simulink model "fcev_model"  (R2023a)
settings: Solver=VariableStepAuto  StartTime=0.0  StopTime=2474  RelTol=1e-3
model workspace (MAT data in the model file):
  N_P0 = 3
values from neighbouring files (symbols this model uses):
  drive_Ki = 1    [fcev_model_parameters.m]
  drive_Kp = 20    [fcev_model_parameters.m]
  env_ambtemp_C = 25    [fcev_model_parameters.m]
  env_grade = 0    [fcev_model_parameters.m]
  env_windx_mps = 0    [fcev_model_parameters.m]
  mot_gearratio = 3.2    [fcev_model_parameters.m]
  mot_maxtrq_Nm = [85, 85, 85, 80, 70, 55, 30]    [fcev_model_parameters.m]
  mot_rotspd_radps = [0, 100, 200, 300, 400, 500, 600]    [fcev_model_parameters.m]
  mot_tirerad_m = 0.31    [fcev_model_parameters.m]
  tank_engydensH2_MJpkg = 120    [fcev_model_parameters.m]
  tank_fccurr_A = -20    [fcev_model_parameters.m]
  tank_fceff = 0.55    [fcev_model_parameters.m]
  tank_Pstart_bar = 350    [fcev_model_parameters.m]
  tank_Rconst = 4.124    [fcev_model_parameters.m]
  tank_temp_K = 298    [fcev_model_parameters.m]
  tank_vol_L = 7    [fcev_model_parameters.m]
libraries: nesl_utility x7, sdl_lib x6, autolibshared x2, fl_lib x2, autolibdatasheetbattery x1, autolibmappedmotor x1
settings Model: Creator=connl  LastModifiedBy=connl
settings SolverCC: MaxConsecutiveMinStep=5  DaesscMode=Robust  SolverResetMethod=Robust
settings DebuggingCC: AlgebraicLoopMsg=none

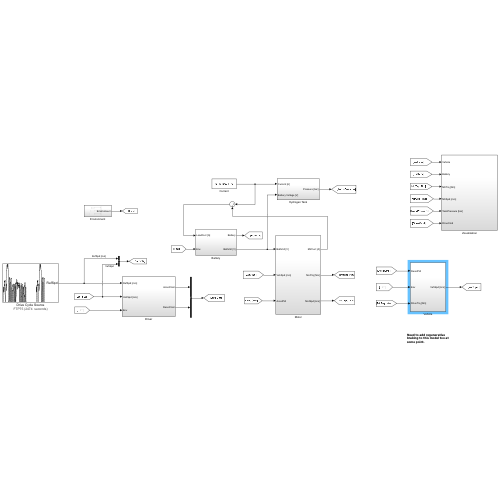
[thumbnail: Simulink's stored preview of the top-level diagram]
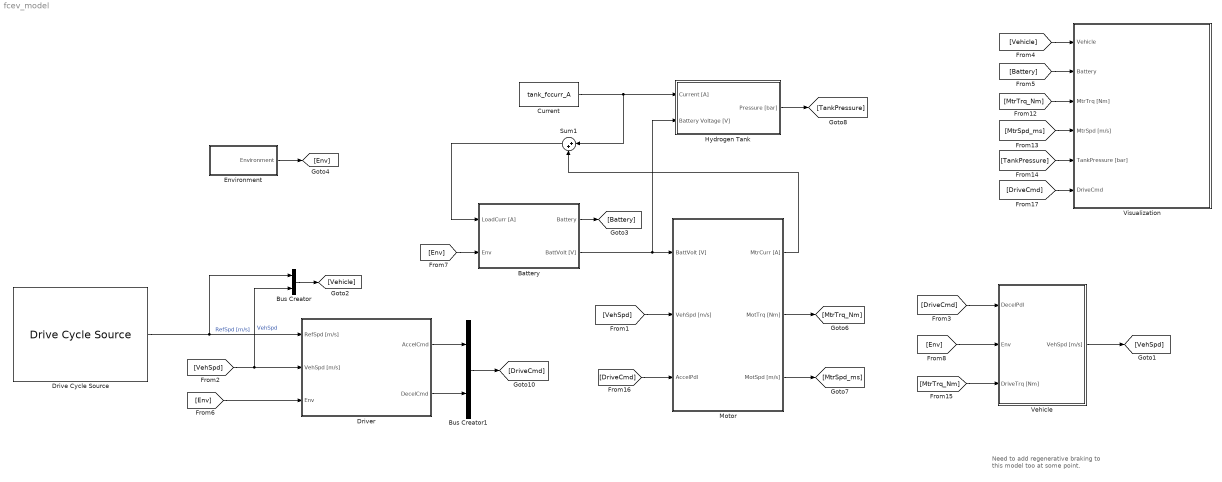
== system fcev_model ==
  note: Need to add regenerative braking to this model too at some point.
  Battery : Subsystem
  Bus Creator : BusCreator  Inputs=2
  Bus Creator1 : BusCreator  Inputs=2
  Current : Constant  Value=tank_fccurr_A
  Drive Cycle Source : autolibshared/Drive Cycle Source  cycleVar=FTP75  fileVar=cycleFTP75.mat  tfinal="2474  seconds"  cycleRepeat=off  outAccPort=off  outGearPort=off  gearList=No gear data  t_wot1=5  xdot_woto=0  xdot_wot1=30  t_wot2=20  xdot_wot2=0  t_wotend=30  srcUnit=m/s  outUnit=m/s  srcAccUnit=m/s/s  outAccUnit=m/s^2  dt=0  aMode=1  faultOption=off  velBnd=2  velBndUnit=mph  inUnit=m/s  timeBnd=1  failOption=off  stopSim=off  maxFaultCnt=10  maxFaultTime=2  maxTotFaultTime=15  traceOption=off  dtTrace=1  traceWindow=10  lastDCname=FTP75  lastOutUnit=mph  lastDT=0  lastTB=1  lastSB=2  forceCalcBound=off
  Driver : Subsystem
  Environment : Subsystem
  Hydrogen Tank : Subsystem
  Motor : Subsystem
  Sum1 : Sum  Inputs=|++
  Vehicle : Subsystem
  Visualization : Subsystem
  wires:
  Drive Cycle Source/1 -> Driver/1(RefSpd [m/s]), Bus Creator/1  "RefSpd [m/s]"
  Battery/2(BattVolt [V]) -> Motor/1(BattVolt [V]), Hydrogen Tank/2(Battery Voltage [V])
  [VehSpd] -> Motor/2(VehSpd [m/s])
  [VehSpd] -> Driver/2(VehSpd [m/s]), Bus Creator/2  "VehSpd"
  [DriveCmd] -> Vehicle/1(DecelPdl)
  Vehicle/1(VehSpd [m/s]) -> [VehSpd]
  Bus Creator/1 -> [Vehicle]
  [Vehicle] -> Visualization/1(Vehicle)
  [Battery] -> Visualization/2(Battery)
  Environment/1(Environment) -> [Env]
  Battery/1(Battery) -> [Battery]
  Driver/2(DecelCmd) -> Bus Creator1/2
  [Env] -> Battery/2(Env)
  [Env] -> Driver/3(Env)
  [Env] -> Vehicle/2(Env)
  Motor/3(MotSpd [m/s]) -> [MtrSpd_ms]
  [MtrTrq_Nm] -> Visualization/3(MtrTrq [Nm])
  [MtrSpd_ms] -> Visualization/4(MtrSpd [m/s])
  Current/1 -> Hydrogen Tank/1(Current [A]), Sum1/1
  Motor/1(MtrCurr [A]) -> Sum1/2
  Sum1/1 -> Battery/1(LoadCurr [A])
  Hydrogen Tank/1(Pressure [bar]) -> [TankPressure]
  [TankPressure] -> Visualization/5(TankPressure [bar])
  Motor/2(MotTrq [Nm]) -> [MtrTrq_Nm]
  [MtrTrq_Nm] -> Vehicle/3(DriveTrq [Nm])
  Driver/1(AccelCmd) -> Bus Creator1/1
  [DriveCmd] -> Motor/3(AccelPdl)
  Bus Creator1/1 -> [DriveCmd]
  [DriveCmd] -> Visualization/6(DriveCmd)

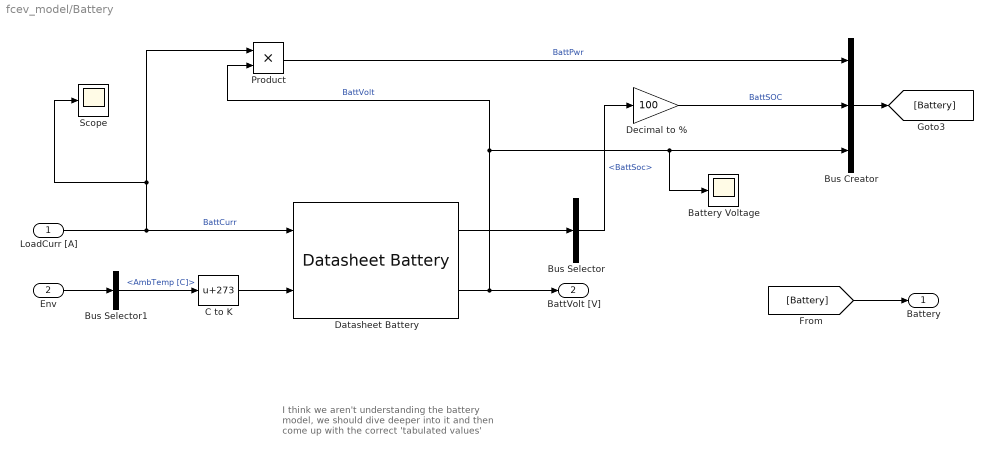
== system fcev_model/Battery ==
  note: I think we aren't understanding the battery model, we should dive deeper into it and then come up with the correct 'tabulated values'
  LoadCurr [A] : Inport
  Env : Inport  Port=2
  Battery Voltage : Scope
  Bus Creator : BusCreator  Inputs=3
  Bus Selector : BusSelector  OutputSignals=BattSoc
  Bus Selector1 : BusSelector  OutputSignals=AmbTemp [C]
  C to K : Bias  Bias=273  SaturateOnIntegerOverflow=off
  Datasheet Battery : autolibdatasheetbattery/Datasheet Battery  CapacityCtrl=Parameter  OutputVlt=Unfiltered  BattChargeMax=batt_ChargeMax_Ah  Em=batt_Em_V  CapLUTBp=batt_CapLUTBp  RInt=batt_RInt  BattTempBp=batt_TempBp_K  CapSOCBp=batt_CapSOCBp  Ns=batt_Ns  Np=batt_Np  BattCapInit=batt_CapInit_Ah  Tc=1/1000  Vinit=4.221  RefBlkName='autolibdatasheetbattery/Datasheet Battery'
  Decimal to % : Gain  Gain=100
  Product : Product
  Scope : Scope
  Battery : Outport
  BattVolt [V] : Outport  Port=2
  wires:
  C to K/1 -> Datasheet Battery/2
  Datasheet Battery/1 -> Bus Selector/1
  Bus Selector/1 -> Decimal to %/1  "<BattSoc>"
  Decimal to %/1 -> Bus Creator/2  "BattSOC"
  Datasheet Battery/2 -> BattVolt [V]/1, Product/2, Bus Creator/3, Battery Voltage/1  "BattVolt"
  [Battery] -> Battery/1
  Env/1 -> Bus Selector1/1
  Bus Selector1/1 -> C to K/1  "<AmbTemp [C]>"
  Product/1 -> Bus Creator/1  "BattPwr"
  LoadCurr [A]/1 -> Scope/1, Product/1, Datasheet Battery/1  "BattCurr"
  Bus Creator/1 -> [Battery]

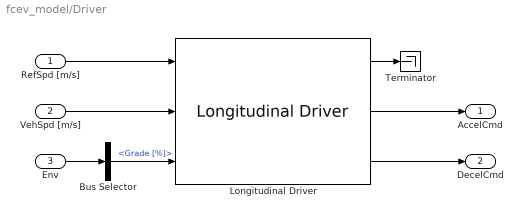
== system fcev_model/Driver ==
  RefSpd [m/s] : Inport
  VehSpd [m/s] : Inport  Port=2
  Env : Inport  Port=3
  Bus Selector : BusSelector  OutputSignals=Grade [%]
  Longitudinal Driver : autolibshared/Longitudinal Driver  extAccelOvr=off  extDecelOvr=off  extAccelHld=off  extDecelHld=off  extAccelZero=off  extDecelZero=off  cntrlType=PI  shftType=None  velUnits=m/s  gearOut=off  Kp=drive_Kp  Ki=drive_Ki  Kff=drive_Kff  Kg=drive_Kg  VehVelVec=[0 100]  KffVec=[.1 .1]  KpVec=[10 10]  KiVec=[5 5]  KgVec=[0 0]  m=1500  Kpt=3000  tau=.1  L=2  aR=200  bR=2.5  cR=.5  g=9.81  vnom=drive_vnom  Kaw=drive_Kaw  tauerr=drive_tauerr  tauPt=2  GearInit=0  tShift=.1  pdlVec=[0.1 0.4 0.5 0.9]  upShftTbl=[-1 12.9375 26.4375 39.9375 51.18749999999999 62.4375 72.84375 83.25;-1 16.3125 29.8125 43.3125 54.5624 65.8125 76.78125 87.75;-1 19.6875 33.1875 46.68749999999999 57.9375 69.1875 80.71875 92.25;-1 33 52.5 77.25 100.5 138.75 161.875 185]  dwnShftTbl=[1 9.5625 23.0625 36.5625 47.8125 59.0625 68.90625 78.75;1 12.9375 26.4375 39.9375 51.18749999999999 62.4375 72.84375 83.25;1 16.3125 29.8125 43.3125 54.562499 65.8125 76.78125 87.75;1 19.6875 33.1875 46.68749999999999 57.9375 69.1875 80.71875 92.25]  tClutch=.5  tRev=.5  tPark=120  aMode=1  UpGearVec="[0  1  2  3  4  5  6  7]"  DownGearVec="[1  2  3  4  5  6  7  8]"
  Terminator : Terminator
  AccelCmd : Outport
  DecelCmd : Outport  Port=2
  wires:
  VehSpd [m/s]/1 -> Longitudinal Driver/2
  Longitudinal Driver/2 -> AccelCmd/1
  RefSpd [m/s]/1 -> Longitudinal Driver/1
  Bus Selector/1 -> Longitudinal Driver/3  "<Grade [%]>"
  Env/1 -> Bus Selector/1
  Longitudinal Driver/3 -> DecelCmd/1
  Longitudinal Driver/1 -> Terminator/1

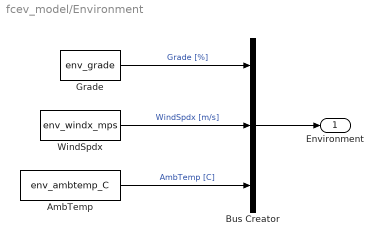
== system fcev_model/Environment ==
  AmbTemp : Constant  Value=env_ambtemp_C
  Bus Creator : BusCreator  Inputs=3
  Grade : Constant  Value=env_grade
  WindSpdx : Constant  Value=env_windx_mps
  Environment : Outport
  wires:
  Grade/1 -> Bus Creator/1  "Grade [%]"
  WindSpdx/1 -> Bus Creator/2  "WindSpdx [m/s]"
  AmbTemp/1 -> Bus Creator/3  "AmbTemp [C]"
  Bus Creator/1 -> Environment/1

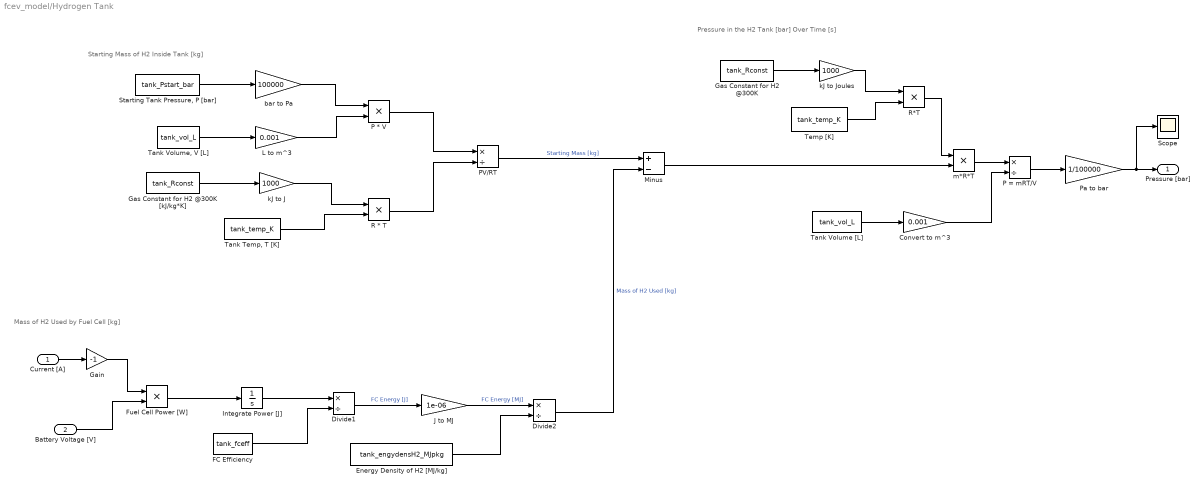
== system fcev_model/Hydrogen Tank ==
  note: Pressure in the H2 Tank [bar] Over Time [s]
  note: Starting Mass of H2 Inside Tank [kg]
  note: Mass of H2 Used by Fuel Cell [kg]
  Current [A] : Inport
  Battery Voltage [V] : Inport  Port=2
  Convert to m^3 : Gain  Gain=0.001
  Divide1 : Product  Inputs=*/
  Divide2 : Product  Inputs=*/
  Energy Density of H2 [MJ/kg] : Constant  Value=tank_engydensH2_MJpkg
  FC Efficiency : Constant  Value=tank_fceff
  Fuel Cell Power [W] : Product
  Gain : Gain  Gain=-1
  Gas Constant for H2 @300K : Constant  Value=tank_Rconst
  Gas Constant for H2 @300K [kJ/kg*K] : Constant  Value=tank_Rconst
  Integrate Power [J] : Integrator
  J to MJ : Gain  Gain=1e-06
  L to m^3 : Gain  Gain=0.001
  Minus : Sum  Inputs=+-
  P * V : Product
  P = mRT/V : Product  Inputs=*/
  PV/RT : Product  Inputs=*/
  Pa to bar : Gain  Gain=1/100000
  R * T : Product
  R*T : Product
  Scope : Scope
  "Starting Tank Pressure, P [bar]" : Constant  Value=tank_Pstart_bar
  "Tank Temp, T [K]" : Constant  Value=tank_temp_K
  Tank Volume [L] : Constant  Value=tank_vol_L
  "Tank Volume, V [L]" : Constant  Value=tank_vol_L
  Temp [K] : Constant  Value=tank_temp_K
  bar to Pa : Gain  Gain=100000
  kJ to J : Gain  Gain=1000
  kJ to Joules : Gain  Gain=1000
  m*R*T : Product
  Pressure [bar] : Outport
  wires:
  P * V/1 -> PV/RT/1
  bar to Pa/1 -> P * V/1
  Pa to bar/1 -> Pressure [bar]/1, Scope/1
  Divide1/1 -> J to MJ/1  "FC Energy [J]"
  PV/RT/1 -> Minus/1  "Starting Mass [kg]"
  Minus/1 -> m*R*T/2
  Gas Constant for H2 @300K/1 -> kJ to Joules/1
  Temp [K]/1 -> R*T/2
  Integrate Power [J]/1 -> Divide1/1
  Gas Constant for H2 @300K [kJ/kg*K]/1 -> kJ to J/1
  R*T/1 -> m*R*T/1
  "Tank Temp, T [K]"/1 -> R * T/2
  Divide2/1 -> Minus/2  "Mass of H2 Used [kg]"
  R * T/1 -> PV/RT/2
  kJ to J/1 -> R * T/1
  FC Efficiency/1 -> Divide1/2
  P = mRT/V/1 -> Pa to bar/1
  Tank Volume [L]/1 -> Convert to m^3/1
  Battery Voltage [V]/1 -> Fuel Cell Power [W]/2
  Convert to m^3/1 -> P = mRT/V/2
  Energy Density of H2 [MJ/kg]/1 -> Divide2/2
  kJ to Joules/1 -> R*T/1
  Fuel Cell Power [W]/1 -> Integrate Power [J]/1
  "Tank Volume, V [L]"/1 -> L to m^3/1
  "Starting Tank Pressure, P [bar]"/1 -> bar to Pa/1
  L to m^3/1 -> P * V/2
  J to MJ/1 -> Divide2/1  "FC Energy [MJ]"
  m*R*T/1 -> P = mRT/V/1
  Current [A]/1 -> Gain/1
  Gain/1 -> Fuel Cell Power [W]/1

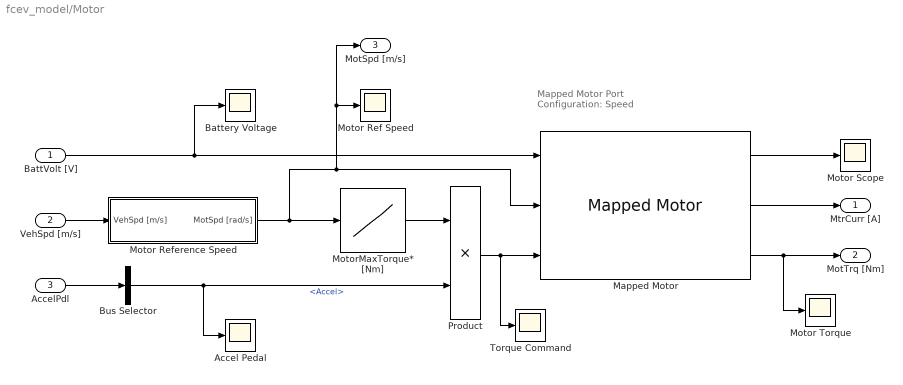
== system fcev_model/Motor ==
  note: Mapped Motor
      | Port Configuration: Speed
  BattVolt [V] : Inport
  VehSpd [m/s] : Inport  Port=2
  AccelPdl : Inport  Port=3
  Accel Pedal : Scope
  Battery Voltage : Scope
  Bus Selector : BusSelector  OutputSignals=Accel
  Mapped Motor : autolibmappedmotor/Mapped Motor  port_config=Speed  param_by=Tabulated torque-speed envelope  w_t=mot_rotspd_radps  T_t=mot_maxtrq_Nm  torque_max=110  power_max=21000  Tc=mot_Tc_s  param_loss=Single efficiency measurement  eff=90  w_eff=400  T_eff=55  Piron=0  Pbase=0  w_eff_bp=[-800 -400 0 400 800]  T_eff_bp=[0 0.03 0.06 0.09]  Temp_eff_bp=[233.15 293.15 373.15]  losses_table=[1.49 1.67 2.21 3.10; 0.42 0.69 1.14 2.03; 0.06 0.24 0.78 1.68; 0.42 0.69 1.14 2.03; 1.49 1.67 2.21 3.10]  losses_table_3d=cat(3,[1.49 1.67 2.21 3.10; 0.42 0.69 1.14 2.03; 0.06 0.24 0.78 1.68; 0.42 0.69 1.14 2.03; 1.49 1.67 2.21 3.10],[1.49 1.67 2.21 3.10; 0.42 0.69 1.14 2.03; 0.06 0.24 0.78 1.68; 0.42 0.69 1.14 2.03; 1.49 1.67 2.21 3.10],[1.49 1.67 2.21 3.10; 0.42 0.69 1.14 2.03; 0.06 0.24 0.78 1.68; 0.42 0.69 1.14 2.03; 1.49 1.67 2.21 3.10])  efficiency_table=[95 95 95 95; 95 95 95 95; 95 95 95 95; 95 95 95 95; 95 95 95 95]  efficiency_table_3d=cat(3,[95 95 95 95; 95 95 95 95; 95 95 95 95; 95 95 95 95; 95 95 95 95],[95 95 95 95; 95 95 95 95; 95 95 95 95; 95 95 95 95; 95 95 95 95],[95 95 95 95; 95 95 95 95; 95 95 95 95; 95 95 95 95; 95 95 95 95])  J=5e-6  b=1e-5  omega_o=0  T_t_extended=[30 55 70 80 85 85 85 85 85 80 70 55 30]  w_t_extended=[-600 -500 -400 -300 -200 -100 0 100 200 300 400 500 600]  KLossIron=0  KLossCopper=0.80808  x_w_eff_vec=[-8000 -4000 0 4000 8000]  x_T_eff_vec=[-0.09 -0.06 -0.03 0 0.03 0.06 0.09]  x_tmp_eff_vec=[-0.09 -0.06 -0.03 0 0.03 0.06 0.09]  x_losses_mat=[3.1 2.21 1.67 1.49 1.67 2.21 3.1;2.03 1.14 0.69 0.42 0.69 1.14 2.03;1.68 0.78 0.24 0.06 0.24 0.78 1.68;2.03 1.14 0.69 0.42 0.69 1.14 2.03;3.1 2.21 1.67 1.49 1.67 2.21 3.1]  x_losses_mat_3d=[37.8947368421052 25.2631578947368 12.6315789473684 0 12 24 36;18.9473684210526 12.6315789473684 6.3157894736842 0 5.99999999999999 12 18;0 0 0 0 0 0 0;18 12 5.99999999999999 0 6.3157894736842 12.6315789473684 18.9473684210526;36 24 12 0 12.6315789473684 25.2631578947368 37.8947368421052]  CalLossMapData={}  CalLossWithTempMapData={}  aMode=1  RefBlkName='autolibmappedmotor/Mapped Motor'
      settings: LibrarySourceBlock=autolibemachines/Mapped Motor
  Motor Ref Speed : Scope
  Motor Reference Speed : Subsystem
  Motor Scope : Scope
  Motor Torque : Scope
  MotorMaxTorque* [Nm] : Lookup_n-D  NumberOfTableDimensions=1  BreakpointsForDimension1=mot_rotspd_radps  Table=mot_maxtrq_Nm  InternalRulePriority=Speed  RndMeth=Simplest
  Product : Product
  Torque Command : Scope
  MtrCurr [A] : Outport
  MotTrq [Nm] : Outport  Port=2
  MotSpd [m/s] : Outport  Port=3
  wires:
  VehSpd [m/s]/1 -> Motor Reference Speed/1(VehSpd [m/s])
  MotorMaxTorque* [Nm]/1 -> Product/1
  Product/1 -> Torque Command/1, Mapped Motor/3
  BattVolt [V]/1 -> Battery Voltage/1, Mapped Motor/1
  Mapped Motor/2 -> MtrCurr [A]/1
  Mapped Motor/3 -> Motor Torque/1, MotTrq [Nm]/1
  Motor Reference Speed/1(MotSpd [rad/s]) -> Mapped Motor/2, MotSpd [m/s]/1, Motor Ref Speed/1, MotorMaxTorque* [Nm]/1
  Mapped Motor/1 -> Motor Scope/1
  AccelPdl/1 -> Bus Selector/1
  Bus Selector/1 -> Accel Pedal/1, Product/2  "<Accel>"

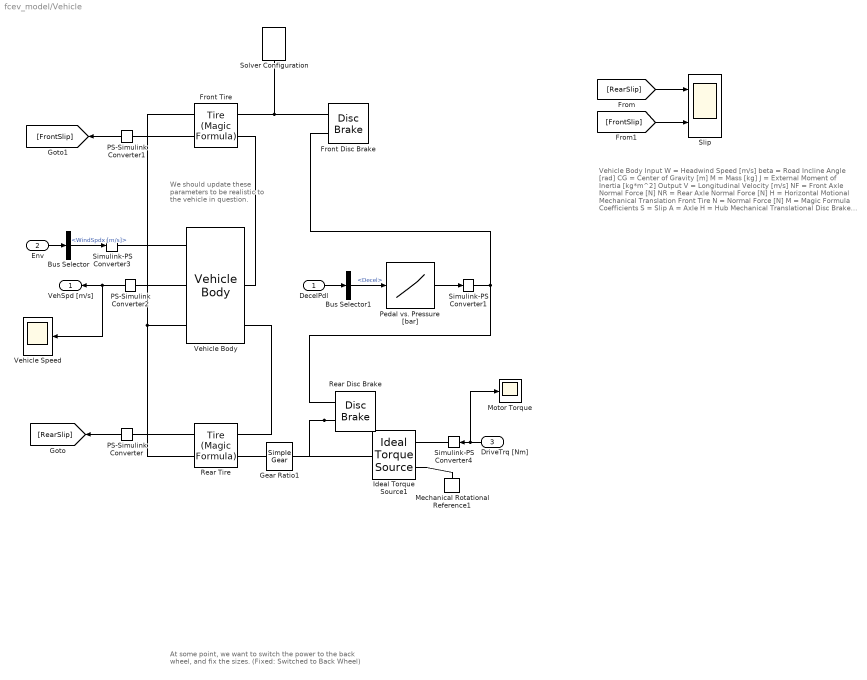
== system fcev_model/Vehicle ==
  note: We should update these parameters to be realistic to the vehicle in question.
  note: Vehicle Body
      | Input
      | W = Headwind Speed [m/s]
      | beta = Road Incline Angle [rad]
      | CG = Center of Gravity [m]
      | M = Mass [kg]
      | J = External Moment of Inertia [kg*m^2]
      |
      | Output
      | V = Longitudinal Velocity [m/s]
      | NF = Front Axle Normal Force [N]
      | NR = Rear Axle Normal Force [N]
      | H = Horizontal Motional Mechanical Translation
      |
      | Front Tire
      | N = Normal Force [N]
      | M = Magic Formula Coefficients
      | S = Slip
      | A = Axle
      | H = Hub Mechanical Translational
      |
      | Disc Brake
      | P = Cylinder Pressure [bars]
      | S = Shaft Rotational Mechanical
      |
      | Ideal Torque Source
      | S = Control Signal [Nm]
      | C = Case Mechanical Rotational with the Source Reference Point
      | R = Rod Mechanical Rotational Port with the Source Moving Part
  note: At some point, we want to switch the power to the back wheel, and fix the sizes.
      | (Fixed: Switched to Back Wheel)
  DecelPdl : Inport
  Env : Inport  Port=2
  DriveTrq [Nm] : Inport  Port=3
  Bus Selector : BusSelector  OutputSignals=WindSpdx [m/s]
  Bus Selector1 : BusSelector  OutputSignals=Decel
  Front Disc Brake : sdl_lib/Brakes & Detents/Rotational/Disc Brake  r_mean=veh_brake_padrad_m m  bore=veh_brakecylbore_m m  n_pads=veh_brakepadnum  thermal_port=simscape.enum.thermaleffects.omit  mu_static=0.1  mu_coulomb=0.1  temperature_TLU=[280, 300, 320] K  mu_static_TLU=[.9, .8, .7]  mu_coulomb_TLU=[.8, .7, .6]  brkwy_vel=0.1 rad/s  visc_coef=0.001 N*m/(rad/s)  enable_faults=simscape.enum.onoff.off  faulted_pressure=0 bar  external_fault=simscape.enum.onoff.off  temporal_fault=simscape.enum.onoff.off  fault_time=5 s  report_fault=simscape.enum.assert.action.none  thermal_mass=50 kJ/K  temperature_specify=off  temperature_priority=High  temperature=300 K  temperature_nominal_specify=off  temperature_nominal_unit=K  temperature_nominal_value=1
  Front Tire : sdl_lib/Tires & Vehicles/Tire (Magic Formula)  parameterization=sdl.enum.magic_tire_model.peak  F_z1=veh_tirevertload_N N  F_x1=veh_tirelongload_N N  kappa1=6  B_m=10  C_m=1.9  D_m=1  E_m=0.97  fz0=4e+3 N  p_Cx=1.685  p_Dx=[ 1.21 -0.037 ]  p_Ex=[ 0.344 0.095 -0.02 0 ]  p_Kx=[ 21.51 -0.163 0.245 ]  p_Hx=[ -0.002 0.002 ]  p_Vx=[ 0 0 ]  rolling_radius_model=sdl.enum.RollingRadiusParameterization.Constant  r_e=mot_tirerad_m m  r_0=0.3 m  breff=8.39  dreff=0.26  freff=0.074  q_re0=0.99  q_v1=0.008  longvl=17 m/s  cz=5e5 N/m  model_resistance=1  resistance_model=1  coeff=0.015  p_tire=250e3 Pa  alpha=-0.003  beta=0.97  coeff_a=84e-4  coeff_b=6.2e-4 s/m  coeff_c=1.6e-4 s^2/m^2  p_tire0=240e3 Pa  fz0_resistance=4000 N  vH0=16 m/s  q_Sy=[.0082, 0, .0014, .001, 0, 0, 1.08, -.5]  v_thr=1e-3 m/s  enable_scaling_coefficients=false  lfzO=1  lcx=1  lmux=1  lex=1  lkx=1  lhx=1  lvx=1  lmy=1  model_compliance=0  stiffness=1e+6 N/m  damping=1000 N/(m/s)  model_inertia=1  inertia=5 kg*m^2  initial_velocity=0 rad/s  vxlow=0.1 m/s  v_tr_thr=0.1*(0.1) m/s  kpumin=-1e5  kpumax=1e5
  Gear Ratio1 : sdl_lib/Gears/Simple Gear  ratio=1/mot_gearratio  rotation_direction=sdl.enum.shaftOutputDirection.same  friction_model=sdl.enum.gear_efficiencies_load.off  T_noload=0.1 N*m  T_nom=5 N*m  efficiency_nom=0.8  efficiency=0.8  temperature_TLU=[280, 300, 320] K  load_TLU=[1, 5, 10] N*m  efficiency_TLU=[.95, .9, .85]  efficiency_TLU2=[.85, .8, .75; .95, .9, .85; .85, .8, .7]  w_thr=0.01 rad/s  pwr_thr=0.001 W  enable_backlash=false  hardstop_model=simscape.enum.hardstop.smooth  backlash_distance=1e-3 mm  r_base=0.1 m  transition=1e-4 mm  backlash_stiffness=1e6 N/m  backlash_damping=1e3 N*s/m  coeff_rest=0.7  v_tol=0.001 m/s  f_tol=0.001 N  mu_visc=[0, 0] N*m*s/rad  enable_faults=simscape.enum.onoff.off  efficiency_fault=0.05  external_fault=simscape.enum.onoff.off  temporal_fault=simscape.enum.onoff.off  fault_time=5 s  fault_angles=pi / 12 rad  report_fault=simscape.enum.assert.action.none  thermal_mass=50 J/K  temperature_specify=off  temperature_priority=High  temperature=300 K  temperature_nominal_specify=off  temperature_nominal_unit=K  temperature_nominal_value=1  x_backlash_specify=off  x_backlash_priority=None  x_backlash=0 mm  x_backlash_nominal_specify=off  x_backlash_nominal_unit=mm  x_backlash_nominal_value=1  f_hardstop_specify=off  f_hardstop_priority=None  f_hardstop=0 N  f_hardstop_nominal_specify=off  f_hardstop_nominal_unit=N  f_hardstop_nominal_value=1  v_backlash_specify=off  v_backlash_priority=None  v_backlash=0 m/s  v_backlash_nominal_specify=off  v_backlash_nominal_unit=m/s  v_backlash_nominal_value=1
  Ideal Torque Source1 : fl_lib/Mechanical/Mechanical Sources/Ideal Torque Source
  Mechanical Rotational Reference1 : fl_lib/Mechanical/Rotational Elements/Mechanical Rotational Reference
  Motor Torque : Scope
  PS-Simulink Converter : nesl_utility/PS-Simulink Converter  PhysicalDomain=network_engine_domain  SubClassName=ps_output  LeftPortType=input  RightPortType=output  PseudoPeriodic=off  Frequencies=[]  VectorFormat=inherit  Unit=inherit  AffineConversion=off
  PS-Simulink Converter1 : nesl_utility/PS-Simulink Converter  PhysicalDomain=network_engine_domain  SubClassName=ps_output  LeftPortType=input  RightPortType=output  PseudoPeriodic=off  Frequencies=[]  VectorFormat=inherit  Unit=inherit  AffineConversion=off
  PS-Simulink Converter2 : nesl_utility/PS-Simulink Converter  PhysicalDomain=network_engine_domain  SubClassName=ps_output  LeftPortType=input  RightPortType=output  PseudoPeriodic=off  Frequencies=[]  VectorFormat=inherit  Unit=m/s  AffineConversion=off
  Pedal vs. Pressure [bar] : Lookup_n-D  NumberOfTableDimensions=1  BreakpointsForDimension1=[-5:5]  Table=tanh([-5:5])  InternalRulePriority=Speed  RndMeth=Simplest
  Rear Disc Brake : sdl_lib/Brakes & Detents/Rotational/Disc Brake  r_mean=veh_brake_padrad_m m  bore=veh_brakecylbore_m m  n_pads=veh_brakepadnum  thermal_port=simscape.enum.thermaleffects.omit  mu_static=0.1  mu_coulomb=0.1  temperature_TLU=[280, 300, 320] K  mu_static_TLU=[.9, .8, .7]  mu_coulomb_TLU=[.8, .7, .6]  brkwy_vel=0.1 rad/s  visc_coef=0.001 N*m/(rad/s)  enable_faults=simscape.enum.onoff.off  faulted_pressure=0 bar  external_fault=simscape.enum.onoff.off  temporal_fault=simscape.enum.onoff.off  fault_time=5 s  report_fault=simscape.enum.assert.action.none  thermal_mass=50 kJ/K  temperature_specify=off  temperature_priority=High  temperature=300 K  temperature_nominal_specify=off  temperature_nominal_unit=K  temperature_nominal_value=1
  Rear Tire : sdl_lib/Tires & Vehicles/Tire (Magic Formula)  parameterization=1  F_z1=veh_tirevertload_N N  F_x1=veh_tirelongload_N N  kappa1=6  B_m=10  C_m=1.9  D_m=1  E_m=0.97  fz0=4e+3 N  p_Cx=1.685  p_Dx=[ 1.21 -0.037 ]  p_Ex=[ 0.344 0.095 -0.02 0 ]  p_Kx=[ 21.51 -0.163 0.245 ]  p_Hx=[ -0.002 0.002 ]  p_Vx=[ 0 0 ]  rolling_radius_model=sdl.enum.RollingRadiusParameterization.Constant  r_e=mot_tirerad_m m  r_0=0.3 m  breff=8.39  dreff=0.26  freff=0.074  q_re0=0.99  q_v1=0.008  longvl=17 m/s  cz=5e5 N/m  model_resistance=1  resistance_model=1  coeff=0.015  p_tire=250e3 Pa  alpha=-0.003  beta=0.97  coeff_a=84e-4  coeff_b=6.2e-4 s/m  coeff_c=1.6e-4 s^2/m^2  p_tire0=240e3 Pa  fz0_resistance=4000 N  vH0=16 m/s  q_Sy=[.0082, 0, .0014, .001, 0, 0, 1.08, -.5]  v_thr=1e-3 m/s  enable_scaling_coefficients=false  lfzO=1  lcx=1  lmux=1  lex=1  lkx=1  lhx=1  lvx=1  lmy=1  model_compliance=0  stiffness=1e+6 N/m  damping=1000 N/(m/s)  model_inertia=1  inertia=5 kg*m^2  initial_velocity=0 rad/s  vxlow=0.1 m/s  v_tr_thr=0.1*(0.1) m/s  kpumin=-1e5  kpumax=1e5
  Simulink-PS Converter1 : nesl_utility/Simulink-PS Converter  PhysicalDomain=network_engine_domain  SubClassName=ps_input  LeftPortType=input  RightPortType=output  PseudoPeriodic=off  Frequencies=[]  NoiseDistribution=none  NoiseParameters=[]  Unit=bar  AffineConversion=off  FilteringAndDerivatives=provide  SimscapeFilterOrder=1  InputFilterTimeConstant=0.01  UdotUserProvided=0
  Simulink-PS Converter3 : nesl_utility/Simulink-PS Converter  PhysicalDomain=network_engine_domain  SubClassName=ps_input  LeftPortType=input  RightPortType=output  PseudoPeriodic=off  Frequencies=[]  NoiseDistribution=none  NoiseParameters=[]  Unit=m/s  AffineConversion=off  FilteringAndDerivatives=provide  SimscapeFilterOrder=1  InputFilterTimeConstant=0.01  UdotUserProvided=0
  Simulink-PS Converter4 : nesl_utility/Simulink-PS Converter  PhysicalDomain=network_engine_domain  SubClassName=ps_input  LeftPortType=input  RightPortType=output  PseudoPeriodic=off  Frequencies=[]  NoiseDistribution=none  NoiseParameters=[]  Unit=N*m  AffineConversion=off  FilteringAndDerivatives=provide  SimscapeFilterOrder=1  InputFilterTimeConstant=0.01  UdotUserProvided=0
  Slip : Scope  NumInputPorts=2
  Solver Configuration : nesl_utility/Solver Configuration  PhysicalDomain=network_engine_domain  SubClassName=solver  LeftPortType=input  RightPortType=generic  Tones=[]  Harmonics=[]  SimulateNoise=off  Profile=off  UseLocalSampling=off  EnableSwitchedLinearOptims=on  FrequencyDomain=off  UseCCode=off  RelTol=0.001  AbsTol=0.001  MinStep=1e-09  ToWorkspace=off  RevertToSquareIcSolve=off  NumHomotopyIterations=100  PhasorMode=off  PhasorModeNumHarmonics=1  ConsistencySolver=NEWTON_XTOL_AFTER_FTOL  IndexReductionMethod=DerivativeReplacement  DoDC=off  ResidualTolerance=1e-09  ConsistencyTolSource=GLOBAL  ConsistencyAbsTol=0.001  ConsistencyRelTol=0.001  ConsistencyTolFactor=0.001  UseLocalSolver=off  LocalSolverChoice=NE_BACKWARD_EULER_ADVANCER  ResolveIndetEquations=on  FunctionEvalNumThread=1  LocalSolverSampleTime=0.001  DoFixedCost=off  MaxNonlinIter=3  MaxModeIter=2  ComputeImpulses=off  ImpulseIterations=2  LinearAlgebra=auto  LinearAlgebraNumThread=0  EquationFormulation=NE_TIME_EF  DelaysMemoryBudget=1024  AutomaticFiltering=on  FilteringTimeConstant=0.001  PartitionStorageMethod=AS_NEEDED  PartitionMemoryBudget=1024  PartitionMethod=ROBUST
  Vehicle Body : sdl_lib/Tires & Vehicles/Vehicle Body  mass=veh_mass_kg kg  n_w=veh_wheelpaxle  x_f=veh_xCGfront_m m  x_r=veh_xCGrear_m m  y_c=veh_yCG_m m  mass_var=simscape.enum.onoff.off  g=9.81 m/s^2  liftoff_warning=0  area=veh_frontarea_m2 m^2  Cd=veh_dragcoeff  rho=veh_airdens_kgpm3 kg/m^3  model_pitch=simscape.enum.onoff.off  inertia=4000 kg*m^2  suspension_model=1  k_f=1e4 N/m  b_f=1e4 N/(m/s)  k_r=1e4 N/m  b_r=1e4 N/(m/s)  k_f_TLU=[-2000, -1000, 0, 1000, 2000] N  x_f_TLU=[-.4, -.2, 0, .2, .4] m  b_f_TLU=[-200, -100, 0, 100, 200] N  v_f_TLU=[-4, -2, 0, 2, 4] m/s  k_r_TLU=[-2000, -1000, 0, 1000, 2000] N  x_r_TLU=[-.4, -.2, 0, .2, .4] m  b_r_TLU=[-200, -100, 0, 100, 200] N  v_r_TLU=[-4, -2, 0, 2, 4] m/s  interp_method=simscape.enum.interpolation.linear  extrap_method=simscape.enum.extrapolation.linear  model_hardstop=0  upper_bound_f=.25 m  lower_bound_f=-.25 m  stop_k_f=1e6 N/m  stop_b_f=150 N/(m/s)  upper_bound_r=.25 m  lower_bound_r=-.25 m  stop_k_r=1e6 N/m  stop_b_r=150 N/(m/s)  initial_pitch=0 rad  initial_pitch_rate=0 rad/s  v_specify=on  v_priority=High  v=0 m/s  v_nominal_specify=off  v_nominal_unit=m/s  v_nominal_value=1
  Vehicle Speed : Scope
  VehSpd [m/s] : Outport
  wires:
  PS-Simulink Converter/1 -> [RearSlip]
  [RearSlip] -> Slip/1
  PS-Simulink Converter1/1 -> [FrontSlip]
  [FrontSlip] -> Slip/2
  PS-Simulink Converter2/1 -> Vehicle Speed/1, VehSpd [m/s]/1
  Bus Selector/1 -> Simulink-PS Converter3/1  "<WindSpdx [m/s]>"
  Pedal vs. Pressure [bar]/1 -> Simulink-PS Converter1/1
  Env/1 -> Bus Selector/1
  DriveTrq [Nm]/1 -> Motor Torque/1, Simulink-PS Converter4/1
  DecelPdl/1 -> Bus Selector1/1
  Bus Selector1/1 -> Pedal vs. Pressure [bar]/1  "<Decel>"
  connections:
  Rear Tire/RConn1 -- PS-Simulink Converter/LConn1
  Front Tire/RConn1 -- PS-Simulink Converter1/LConn1
  Vehicle Body/LConn1 -- Rear Tire/RConn2 -- Front Tire/RConn2
  Vehicle Body/RConn1 -- Rear Tire/LConn1
  Vehicle Body/RConn2 -- Front Tire/LConn1
  Rear Disc Brake/LConn2 -- Gear Ratio1/RConn1 -- Ideal Torque Source1/LConn1
  Simulink-PS Converter1/RConn1 -- Rear Disc Brake/LConn1 -- Front Disc Brake/LConn1
  Vehicle Body/LConn2 -- PS-Simulink Converter2/LConn1
  Simulink-PS Converter3/RConn1 -- Vehicle Body/LConn3
  Front Disc Brake/LConn2 -- Solver Configuration/RConn1 -- Front Tire/LConn2
  Ideal Torque Source1/RConn2 -- Mechanical Rotational Reference1/LConn1
  Ideal Torque Source1/RConn1 -- Simulink-PS Converter4/RConn1
  Rear Tire/LConn2 -- Gear Ratio1/LConn1

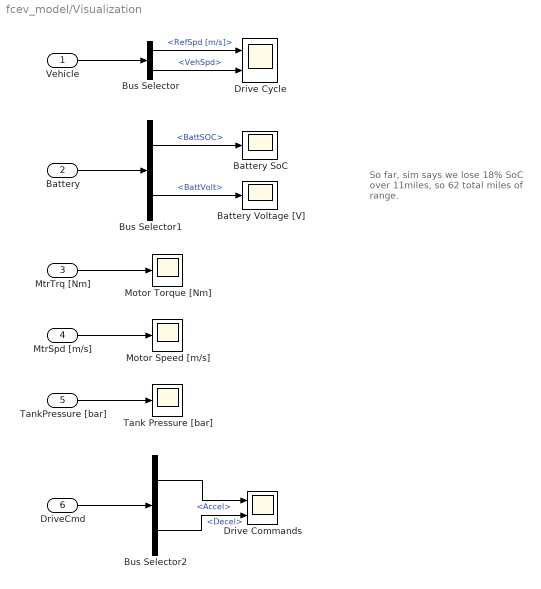
== system fcev_model/Visualization ==
  note: So far, sim says we lose 18% SoC over 11miles, so 62 total miles of range.
  Vehicle : Inport
  Battery : Inport  Port=2
  MtrTrq [Nm] : Inport  Port=3
  MtrSpd [m/s] : Inport  Port=4
  TankPressure [bar] : Inport  Port=5
  DriveCmd : Inport  Port=6
  Battery SoC : Scope
  Battery Voltage [V] : Scope
  Bus Selector : BusSelector  OutputSignals=RefSpd [m/s],VehSpd
  Bus Selector1 : BusSelector  OutputSignals=BattSOC,BattVolt
  Bus Selector2 : BusSelector  OutputSignals=Accel,Decel
  Drive Commands : Scope  NumInputPorts=2
  Drive Cycle : Scope  NumInputPorts=2
  Motor Speed [m/s] : Scope
  Motor Torque [Nm] : Scope
  Tank Pressure [bar] : Scope
  wires:
  Vehicle/1 -> Bus Selector/1
  Battery/1 -> Bus Selector1/1
  Bus Selector/1 -> Drive Cycle/1  "<RefSpd [m/s]>"
  Bus Selector/2 -> Drive Cycle/2  "<VehSpd>"
  Bus Selector1/1 -> Battery SoC/1  "<BattSOC>"
  Bus Selector1/2 -> Battery Voltage [V]/1  "<BattVolt>"
  MtrTrq [Nm]/1 -> Motor Torque [Nm]/1
  MtrSpd [m/s]/1 -> Motor Speed [m/s]/1
  TankPressure [bar]/1 -> Tank Pressure [bar]/1
  DriveCmd/1 -> Bus Selector2/1
  Bus Selector2/1 -> Drive Commands/1  "<Accel>"
  Bus Selector2/2 -> Drive Commands/2  "<Decel>"

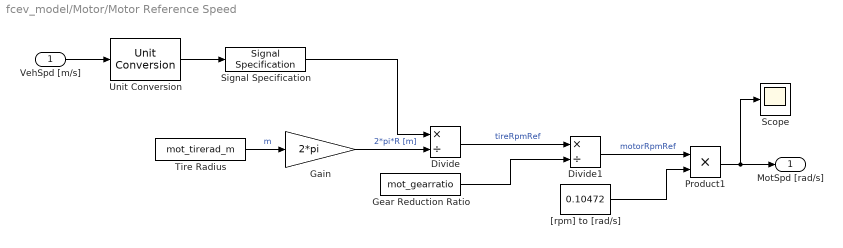
== system fcev_model/Motor/Motor Reference Speed ==
  VehSpd [m/s] : Inport
  Divide : Product  Inputs=*/
  Divide1 : Product  Inputs=*/
  Gain : Gain  Gain=2*pi
  Gear Reduction Ratio : Constant  Value=mot_gearratio
  Product1 : Product
  Scope : Scope
  Signal Specification : SignalSpecification  Unit=m/min
  Tire Radius : Constant  Value=mot_tirerad_m
  Unit Conversion : UnitConversion
  "[rpm] to [rad/s]" : Constant  Value=0.10472
  MotSpd [rad/s] : Outport
  wires:
  VehSpd [m/s]/1 -> Unit Conversion/1
  Divide/1 -> Divide1/1  "tireRpmRef"
  Gain/1 -> Divide/2  "2*pi*R [m]"
  Gear Reduction Ratio/1 -> Divide1/2
  Tire Radius/1 -> Gain/1  "m"
  Product1/1 -> MotSpd [rad/s]/1, Scope/1
  "[rpm] to [rad/s]"/1 -> Product1/2
  Divide1/1 -> Product1/1  "motorRpmRef"
  Signal Specification/1 -> Divide/1
  Unit Conversion/1 -> Signal Specification/1
